simulink model "wheel_dynamics_FL1"  (R2023b)
settings: Solver=VariableStepAuto  StartTime=0.0  StopTime=10.0  RelTol=1e-3
values from neighbouring files (symbols this model uses):
  f0 = 0.009    [Load_Params.m]
  f2 = 6.5e-6    (= 6.5e-06)    [Load_Params.m]
  velstart = 0.01    [Load_Params.m]
undefined symbols (not defined in the file or in its folder): lr, x0
settings Model: Creator=angel  LastModifiedBy=angel

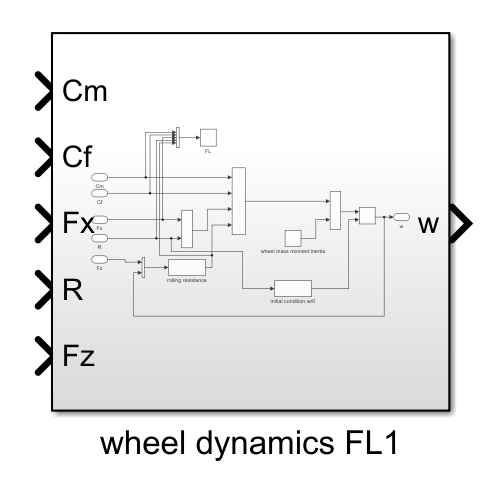
[thumbnail: Simulink's stored preview of the top-level diagram]
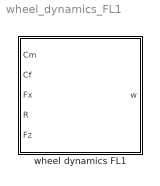
== system wheel_dynamics_FL1 ==
  wheel dynamics FL1 : Subsystem

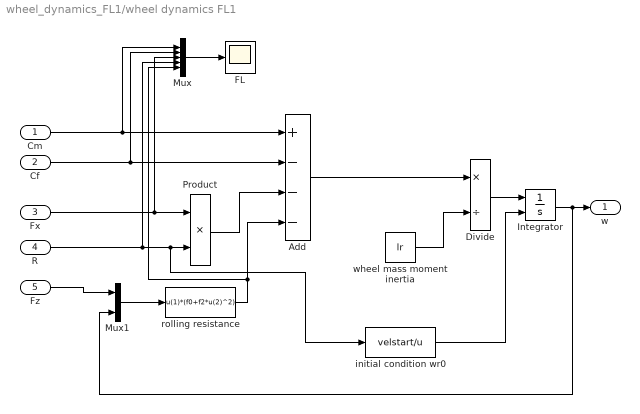
== system wheel_dynamics_FL1/wheel dynamics FL1 ==
  Cm : Inport
  Cf : Inport  Port=2
  Fx : Inport  Port=3
  R : Inport  Port=4
  Fz : Inport  Port=5
  Add : Sum  Inputs=+---
  Divide : Product  Inputs=*/
  FL : Scope
  Integrator : Integrator  InitialConditionSource=external  InitialCondition=x0
  Mux : Mux  Inputs=5
  Mux1 : Mux  Inputs=2
  Product : Product
  initial condition wr0 : MATLABFcn  MATLABFcn=velstart/u
  rolling resistance : MATLABFcn  MATLABFcn=u(1)*(f0+f2*u(2)^2)
  wheel mass moment inertia : Constant  Value=lr
  w : Outport
  wires:
  Cm/1 -> Mux/1, Add/1
  R/1 -> Mux/4, initial condition wr0/1, Product/2
  rolling resistance/1 -> Add/4, Mux/5
  Cf/1 -> Mux/2, Add/2
  Fx/1 -> Mux/3, Product/1
  Product/1 -> Add/3
  Mux/1 -> FL/1
  Add/1 -> Divide/1
  wheel mass moment inertia/1 -> Divide/2
  Divide/1 -> Integrator/1
  initial condition wr0/1 -> Integrator/2
  Integrator/1 -> w/1, Mux1/2
  Fz/1 -> Mux1/1
  Mux1/1 -> rolling resistance/1
